simulink subsystem "HardwareInputs"  (R2019b)
settings: Solver=VariableStepAuto  StartTime=0.0  StopTime=10.0  RelTol=1e-3
undefined symbols (not defined in the file): __PRM__SERIALIZED__DATA__, SubsystemReferenceBlock
libraries: FunctionCallDivider x3
settings Model: Creator=Nick  LastModifiedBy=zacha

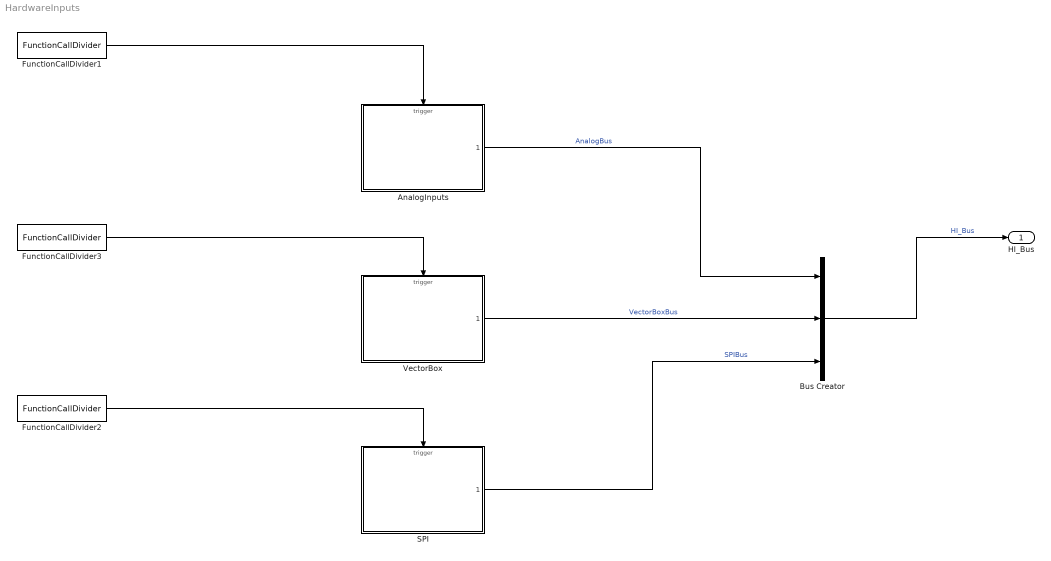
== system HardwareInputs ==
  AnalogInputs : Subsystem  BlockKeywords=__PRM__SERIALIZED__DATA__:SubsystemReferenceBlock  ReferencedSubsystem=HI_AnalogInputs
  Bus Creator : BusCreator  Inputs=3
  FunctionCallDivider1 : FunctionCallDivider/Algroithms/FunctionCallDivider  counts=100
  FunctionCallDivider2 : FunctionCallDivider/Algroithms/FunctionCallDivider  counts=1
  FunctionCallDivider3 : FunctionCallDivider/Algroithms/FunctionCallDivider  counts=1
  SPI : Subsystem  BlockKeywords=__PRM__SERIALIZED__DATA__:SubsystemReferenceBlock  ReferencedSubsystem=HI_SPI
  VectorBox : Subsystem  BlockKeywords=__PRM__SERIALIZED__DATA__:SubsystemReferenceBlock  ReferencedSubsystem=HI_VectorBox
  HI_Bus : Outport
  wires:
  FunctionCallDivider1/1 -> AnalogInputs/Trigger
  Bus Creator/1 -> HI_Bus/1  "HI_Bus"
  AnalogInputs/1 -> Bus Creator/1  "AnalogBus"
  VectorBox/1 -> Bus Creator/2  "VectorBoxBus"
  FunctionCallDivider3/1 -> VectorBox/Trigger
  SPI/1 -> Bus Creator/3  "SPIBus"
  FunctionCallDivider2/1 -> SPI/Trigger
